simulink model "array_and_Darray_doubleRx"  (R2019b)
settings: Solver=VariableStepAuto  StartTime=0.0  StopTime=0.0005  RelTol=1e-3
libraries: fl_lib x54, nesl_utility x34, ee_lib x17, powerlib_meascontrol x5
settings Model: Creator=LRF  LastModifiedBy=LRF

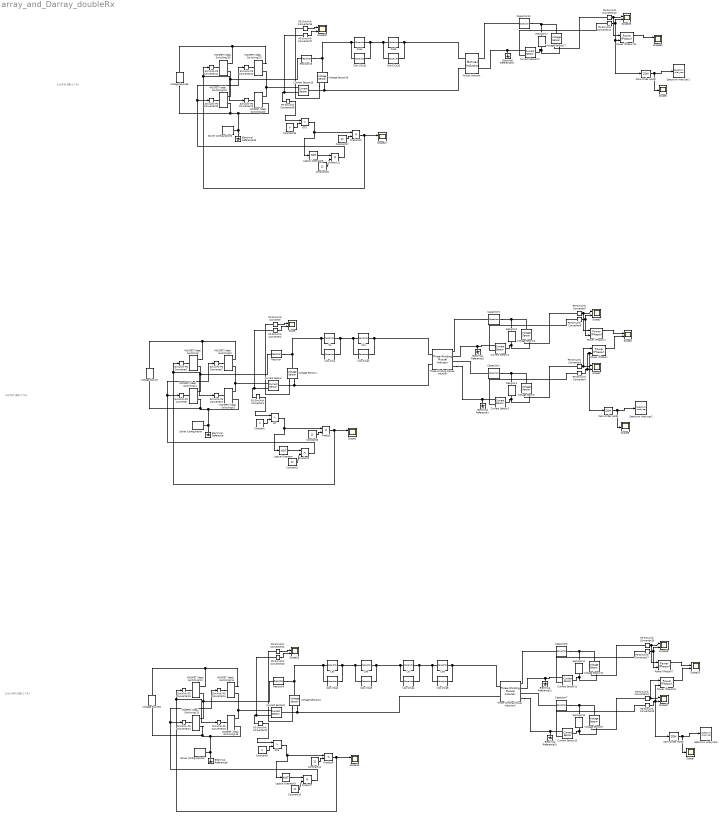
== system array_and_Darray_doubleRx ==
  note: 2x1阵列 搭配 2个Rx
  note: 2x1阵列 搭配 1个Rx
  note: 2x2x1阵列 搭配 2个Rx
  (2/a-1)Ca{,1..5,11..12} (8 alike) : fl_lib/Electrical/Electrical Elements/Capacitor  c=379 pF  r=1e-6 Ohm  g=0 1/Ohm  i_specify=off  i_priority=None  i=0 A  i_nominal_specify=off  i_nominal_unit=A  i_nominal_value=1  v_specify=off  v_priority=None  v=0 V  v_nominal_specify=off  v_nominal_unit=V  v_nominal_value=1  vc_specify=off  vc_priority=High  vc=0 V  vc_nominal_specify=off  vc_nominal_unit=V  vc_nominal_value=1
  Ca{,1,5..8,14..15} (8 alike) : fl_lib/Electrical/Electrical Elements/Capacitor  c=1517 pF  r=1e-6 Ohm  g=0 1/Ohm  i_specify=off  i_priority=None  i=0 A  i_nominal_specify=off  i_nominal_unit=A  i_nominal_value=1  v_specify=off  v_priority=None  v=0 V  v_nominal_specify=off  v_nominal_unit=V  v_nominal_value=1  vc_specify=off  vc_priority=High  vc=0 V  vc_nominal_specify=off  vc_nominal_unit=V  vc_nominal_value=1
  Capacitor{1,3,7..8,12} (5 alike) : fl_lib/Electrical/Electrical Elements/Capacitor  c=1013 pF  r=1e-6 Ohm  g=0 1/Ohm  i_specify=off  i_priority=None  i=0 A  i_nominal_specify=off  i_nominal_unit=A  i_nominal_value=1  v_specify=off  v_priority=None  v=0 V  v_nominal_specify=off  v_nominal_unit=V  v_nominal_value=1  vc_specify=off  vc_priority=High  vc=0 V  vc_nominal_specify=off  vc_nominal_unit=V  vc_nominal_value=1
  Constant : Constant  Value=0
  Constant{1,3,10..11,16..17} (6 alike) : Constant  Value=12
  Constant15 : Constant  Value=0
  Constant9 : Constant  Value=0
  Current Sensor{,1..2,9..11,15,17} (8 alike) : fl_lib/Electrical/Electrical Sensors/Current Sensor
  Electrical Reference{,1..2,9..11,15,17} (8 alike) : fl_lib/Electrical/Electrical Elements/Electrical Reference
  GT : RelationalOperator  Operator=>  OutDataTypeStr=boolean  RndMeth=Simplest
  GT3 : RelationalOperator  Operator=>  OutDataTypeStr=boolean  RndMeth=Simplest
  GT5 : RelationalOperator  Operator=>  OutDataTypeStr=boolean  RndMeth=Simplest
  Logical Operator : Logic  Operator=NOT  AllPortsSameDT=off  OutDataTypeStr=boolean
  Logical Operator3 : Logic  Operator=NOT  AllPortsSameDT=off  OutDataTypeStr=boolean
  Logical Operator5 : Logic  Operator=NOT  AllPortsSameDT=off  OutDataTypeStr=boolean
  MOSFET (Ideal, Switching){,1..3,12..15,20..23} (12 alike) : ee_lib/Semiconductors & Converters/MOSFET (Ideal, Switching)  Rds=0.01 Ohm  Goff=1e-6 1/Ohm  Vth=2 V  diode_param=1  diode_Vf=0.8 V  diode_Ron=0.001 Ohm  diode_Goff=1e-5 1/Ohm  diode_C=50e-9 F  diode_iRM=-235 A  diode_iF=300 A  diode_idot=-50 A/us  diode_trr_param=1  diode_trr_factor=3  diode_trr=15 us  diode_Qrr=1500 s*uA  thermal_loss_option=2  Voff=300 V  Tau=1e-4 s  Tj=[298.15, 398.15] K  Iout_scalar=600 A  Eon_scalar=22.86e-3 J  Eoff_scalar=17.14e-3 J  Von_scalar=2.7 V  Iout_data=[0, 10, 50, 100, 200, 400, 600] A  Eon_data=[0, .29, 1.43, 2.86, 5.71, 13.14, 22.86; 0, .57, 2.63, 5.14, 10.29, 20.57, 30.29] * 1e-3 J  Eoff_data=[0, .21, 1.07, 2.14, 4.29, 9.86, 17.14; 0, .43, 1.97, 3.86, 7.71, 15.43, 22.71] * 1e-3 J  Von_data=[0, 1.1, 1.3, 1.45, 1.75, 2.25, 2.7; 0, 1, 1.15, 1.35, 1.7, 2.35, 3] V
      settings: SourceProductName=Simscape Electrical
  Mutual Inductor : fl_lib/Electrical/Electrical Elements/Mutual Inductor  L1=106.94 uH  L2=100 uH  k=0.1  i1_specify=off  i1_priority=High  i1=0 A  i1_nominal_specify=off  i1_nominal_unit=A  i1_nominal_value=1  i2_specify=off  i2_priority=High  i2=0 A  i2_nominal_specify=off  i2_nominal_unit=A  i2_nominal_value=1  v1_specify=off  v1_priority=None  v1=0 V  v1_nominal_specify=off  v1_nominal_unit=V  v1_nominal_value=1  v2_specify=off  v2_priority=None  v2=0 V  v2_nominal_specify=off  v2_nominal_unit=V  v2_nominal_value=1
      settings: SourceProductName=Simscape  SourceProductBaseCode=SS  InternalSimscapePortConfiguration="{\"Bottom\":[],\"Left\":[{\"id\":\"p1\",\"label\":\"1+\",\"type\":\"foundation.electrical.electrical\"},{\"id\":\"n1\",\"label\":\"1-\",\"type\":\"foundation.electrical.electrical\"}],\"Right\":[{\"id\":\"p2\",\"label\":\"2+\",\"type\":\"foundation.electrical.electrical\"},{\"id\":\"n2\",\"label\":\"2-\",\"type\":\"foundation.electrical.electrical\"}],\"Top\":[]}"
  PS-Simulink Converter{,1..6,21..27,35..37,40..41} (19 alike) : nesl_utility/PS-Simulink Converter  PhysicalDomain=network_engine_domain  SubClassName=ps_output  LeftPortType=input  RightPortType=output  PseudoPeriodic=off  Frequencies=[]  Unit=inherit  AffineConversion=off
  Power (Phasor){,1,6..7,11} (5 alike) : powerlib_meascontrol/Measurements/Power (Phasor)
      settings: SourceProductName=Simscape Electrical  SourceProductBaseCode=PS
  Product{,1,6..7,10..11} (6 alike) : Product
  Resistor : fl_lib/Electrical/Electrical Elements/Resistor  R=0 Ohm  i_specify=off  i_priority=None  i=0 A  i_nominal_specify=off  i_nominal_unit=A  i_nominal_value=1  v_specify=off  v_priority=None  v=0 V  v_nominal_specify=off  v_nominal_unit=V  v_nominal_value=1
  Resistor{1..2,10..11,17} (5 alike) : fl_lib/Electrical/Electrical Elements/Resistor  R=15 Ohm  i_specify=off  i_priority=None  i=0 A  i_nominal_specify=off  i_nominal_unit=A  i_nominal_value=1  v_specify=off  v_priority=None  v=0 V  v_nominal_specify=off  v_nominal_unit=V  v_nominal_value=1
  Resistor15 : fl_lib/Electrical/Electrical Elements/Resistor  R=0 Ohm  i_specify=off  i_priority=None  i=0 A  i_nominal_specify=off  i_nominal_unit=A  i_nominal_value=1  v_specify=off  v_priority=None  v=0 V  v_nominal_specify=off  v_nominal_unit=V  v_nominal_value=1
  Resistor9 : fl_lib/Electrical/Electrical Elements/Resistor  R=0 Ohm  i_specify=off  i_priority=None  i=0 A  i_nominal_specify=off  i_nominal_unit=A  i_nominal_value=1  v_specify=off  v_priority=None  v=0 V  v_nominal_specify=off  v_nominal_unit=V  v_nominal_value=1
  Scope{,1..4,15..19,26..27,29..30} (14 alike) : Scope  NumInputPorts=2
  Scope5 : Scope
  Scope6 : Scope
  Scope7 : Scope
  Simulink-PS Converter{,1..3,12..15,20..23} (12 alike) : nesl_utility/Simulink-PS Converter  PhysicalDomain=network_engine_domain  SubClassName=ps_input  LeftPortType=input  RightPortType=output  PseudoPeriodic=off  Frequencies=[]  NoiseDistribution=none  NoiseParameters=[]  Unit=1  AffineConversion=off  FilteringAndDerivatives=provide  SimscapeFilterOrder=1  InputFilterTimeConstant=0.001  UdotUserProvided=0
  Solver Configuration : nesl_utility/Solver Configuration  PhysicalDomain=network_engine_domain  SubClassName=solver  LeftPortType=input  RightPortType=generic  Tones=[]  Harmonics=[]  SimulateNoise=off  Profile=off  UseLocalSampling=off  EnableSwitchedLinearOptims=on  FrequencyDomain=off  UseCCode=off  RelTol=0.001  AbsTol=1e-06  MinStep=1e-09  ToWorkspace=off  RevertToSquareIcSolve=off  NumHomotopyIterations=100  PhasorMode=off  PhasorModeNumHarmonics=1  DoDC=off  ResidualTolerance=1e-09  UseLocalSolver=off  LocalSolverChoice=NE_BACKWARD_EULER_ADVANCER  LocalSolverSampleTime=0.001  DoFixedCost=off  MaxNonlinIter=3  MaxModeIter=2  LinearAlgebra=auto  EquationFormulation=NE_TIME_EF  DelaysMemoryBudget=1024  AutomaticFiltering=on  FilteringTimeConstant=0.001  PartitionStorageMethod=AS_NEEDED  PartitionMemoryBudget=1024  PartitionMethod=ROBUST
  Solver Configuration3 : nesl_utility/Solver Configuration  PhysicalDomain=network_engine_domain  SubClassName=solver  LeftPortType=input  RightPortType=generic  Tones=[]  Harmonics=[]  SimulateNoise=off  Profile=off  UseLocalSampling=off  EnableSwitchedLinearOptims=on  FrequencyDomain=off  UseCCode=off  RelTol=0.001  AbsTol=1e-06  MinStep=1e-09  ToWorkspace=off  RevertToSquareIcSolve=off  NumHomotopyIterations=100  PhasorMode=off  PhasorModeNumHarmonics=1  DoDC=off  ResidualTolerance=1e-09  UseLocalSolver=off  LocalSolverChoice=NE_BACKWARD_EULER_ADVANCER  LocalSolverSampleTime=0.001  DoFixedCost=off  MaxNonlinIter=3  MaxModeIter=2  LinearAlgebra=auto  EquationFormulation=NE_TIME_EF  DelaysMemoryBudget=1024  AutomaticFiltering=on  FilteringTimeConstant=0.001  PartitionStorageMethod=AS_NEEDED  PartitionMemoryBudget=1024  PartitionMethod=ROBUST
  Solver Configuration5 : nesl_utility/Solver Configuration  PhysicalDomain=network_engine_domain  SubClassName=solver  LeftPortType=input  RightPortType=generic  Tones=[]  Harmonics=[]  SimulateNoise=off  Profile=off  UseLocalSampling=off  EnableSwitchedLinearOptims=on  FrequencyDomain=off  UseCCode=off  RelTol=0.001  AbsTol=1e-06  MinStep=1e-09  ToWorkspace=off  RevertToSquareIcSolve=off  NumHomotopyIterations=100  PhasorMode=off  PhasorModeNumHarmonics=1  DoDC=off  ResidualTolerance=1e-09  UseLocalSolver=off  LocalSolverChoice=NE_BACKWARD_EULER_ADVANCER  LocalSolverSampleTime=0.001  DoFixedCost=off  MaxNonlinIter=3  MaxModeIter=2  LinearAlgebra=auto  EquationFormulation=NE_TIME_EF  DelaysMemoryBudget=1024  AutomaticFiltering=on  FilteringTimeConstant=0.001  PartitionStorageMethod=AS_NEEDED  PartitionMemoryBudget=1024  PartitionMethod=ROBUST
  Spectrum Analyzer1 : SpectrumAnalyzer
  Spectrum Analyzer2 : SpectrumAnalyzer
  Spectrum Analyzer3 : SpectrumAnalyzer
  Three-Winding Mutual Inductor : ee_lib/Passive/Transformers/Three-Winding Mutual Inductor  L1=106.94 uH  L2=100 uH  L3=100 uH  K12=0.1  K13=0.1  K23=0  IC_given=1  IC1=0 A  IC2=0 A  IC3=0 A
      settings: SourceProductName=Simscape Electrical  SourceProductBaseCode=PS  InternalSimscapePortConfiguration="{\"Bottom\":[],\"Left\":[{\"id\":\"p1\",\"label\":\"1+\",\"type\":\"foundation.electrical.electrical\"},{\"id\":\"n1\",\"label\":\"1-\",\"type\":\"foundation.electrical.electrical\"}],\"Right\":[{\"id\":\"p2\",\"label\":\"2+\",\"type\":\"foundation.electrical.electrical\"},{\"id\":\"n2\",\"label\":\"2-\",\"type\":\"foundation.electrical.electrical\"},{\"id\":\"p3\",\"label\":\"3+\",\"type\":\"foundation.electrical.electrical\"},{\"id\":\"n3\",\"label\":\"3-\",\"type\":\"foundation.electrical.electrical\"}],\"Top\":[]}"
  Three-Winding Mutual Inductor3 : ee_lib/Passive/Transformers/Three-Winding Mutual Inductor  L1=213.88 uH  L2=100 uH  L3=100 uH  K12=0.1  K13=0.1  K23=0  IC_given=1  IC1=0 A  IC2=0 A  IC3=0 A
      settings: SourceProductName=Simscape Electrical  SourceProductBaseCode=PS  InternalSimscapePortConfiguration="{\"Bottom\":[],\"Left\":[{\"id\":\"p1\",\"label\":\"1+\",\"type\":\"foundation.electrical.electrical\"},{\"id\":\"n1\",\"label\":\"1-\",\"type\":\"foundation.electrical.electrical\"}],\"Right\":[{\"id\":\"p2\",\"label\":\"2+\",\"type\":\"foundation.electrical.electrical\"},{\"id\":\"n2\",\"label\":\"2-\",\"type\":\"foundation.electrical.electrical\"},{\"id\":\"p3\",\"label\":\"3+\",\"type\":\"foundation.electrical.electrical\"},{\"id\":\"n3\",\"label\":\"3-\",\"type\":\"foundation.electrical.electrical\"}],\"Top\":[]}"
  Voltage Sensor{,1..2,9..11,16..17} (8 alike) : fl_lib/Electrical/Electrical Sensors/Voltage Sensor
  Voltage Source : ee_lib/Sources/Voltage Source  dc_voltage=15 V  ac_voltage=0 V  ac_shift=0 rad  ac_frequency=60 Hz  noise_mode=0  PSD=0 V^2/Hz  repeatability=1  auto_seed=3646982598  user_seed=0  sample_time=1e-3 s  i_specify=off  i_priority=None  i=0 A  i_nominal_specify=off  i_nominal_unit=A  i_nominal_value=1  v_specify=off  v_priority=None  v=0 V  v_nominal_specify=off  v_nominal_unit=V  v_nominal_value=1
      settings: SourceProductName=Simscape Electrical
  Voltage Source3 : ee_lib/Sources/Voltage Source  dc_voltage=15 V  ac_voltage=0 V  ac_shift=0 rad  ac_frequency=60 Hz  noise_mode=0  PSD=0 V^2/Hz  repeatability=1  auto_seed=3181899151  user_seed=0  sample_time=1e-3 s  i_specify=off  i_priority=None  i=0 A  i_nominal_specify=off  i_nominal_unit=A  i_nominal_value=1  v_specify=off  v_priority=None  v=0 V  v_nominal_specify=off  v_nominal_unit=V  v_nominal_value=1
      settings: SourceProductName=Simscape Electrical
  Voltage Source5 : ee_lib/Sources/Voltage Source  dc_voltage=15 V  ac_voltage=0 V  ac_shift=0 rad  ac_frequency=60 Hz  noise_mode=0  PSD=0 V^2/Hz  repeatability=1  auto_seed=2586388248  user_seed=0  sample_time=1e-3 s  i_specify=off  i_priority=None  i=0 A  i_nominal_specify=off  i_nominal_unit=A  i_nominal_value=1  v_specify=off  v_priority=None  v=0 V  v_nominal_specify=off  v_nominal_unit=V  v_nominal_value=1
      settings: SourceProductName=Simscape Electrical
  Zero-Order Hold1 : ZeroOrderHold  SampleTime=1e-7
  Zero-Order Hold2 : ZeroOrderHold  SampleTime=1e-7
  Zero-Order Hold3 : ZeroOrderHold  SampleTime=1e-7
  wires:
  PS-Simulink Converter/1 -> Scope/1
  PS-Simulink Converter2/1 -> Scope/2
  PS-Simulink Converter1/1 -> GT/1
  Constant/1 -> GT/2
  GT/1 -> Logical Operator/1, Product/1
  Product/1 -> Simulink-PS Converter3/1, Simulink-PS Converter1/1, Scope1/1
  Constant3/1 -> Product/2
  Logical Operator/1 -> Product1/1
  Constant1/1 -> Product1/2
  Product1/1 -> Simulink-PS Converter2/1, Simulink-PS Converter/1
  PS-Simulink Converter3/1 -> Power (Phasor)/1, Scope2/1
  PS-Simulink Converter6/1 -> Power (Phasor)1/2, Scope3/2
  PS-Simulink Converter5/1 -> Power (Phasor)1/1, Scope3/1
  Power (Phasor)/1 -> Scope4/2
  Power (Phasor)1/1 -> Scope4/1
  PS-Simulink Converter21/1 -> Scope15/1
  PS-Simulink Converter23/1 -> Scope15/2
  PS-Simulink Converter22/1 -> GT3/1
  PS-Simulink Converter27/1 -> Power (Phasor)7/2, Scope18/2
  Power (Phasor)6/1 -> Scope19/2
  GT3/1 -> Logical Operator3/1, Product6/1
  PS-Simulink Converter24/1 -> Power (Phasor)6/1, Scope17/1
  Product6/1 -> Simulink-PS Converter15/1, Simulink-PS Converter13/1, Scope16/1
  Logical Operator3/1 -> Product7/1
  Product7/1 -> Simulink-PS Converter14/1, Simulink-PS Converter12/1
  Constant9/1 -> GT3/2
  Power (Phasor)7/1 -> Scope19/1
  Constant11/1 -> Product6/2
  Constant10/1 -> Product7/2
  PS-Simulink Converter26/1 -> Power (Phasor)7/1, Scope18/1
  PS-Simulink Converter35/1 -> Scope26/1
  PS-Simulink Converter37/1 -> Scope26/2
  PS-Simulink Converter36/1 -> GT5/1
  GT5/1 -> Logical Operator5/1, Product10/1
  Product10/1 -> Simulink-PS Converter23/1, Simulink-PS Converter21/1, Scope27/1
  Logical Operator5/1 -> Product11/1
  Product11/1 -> Simulink-PS Converter22/1, Simulink-PS Converter20/1
  Constant15/1 -> GT5/2
  Power (Phasor)11/1 -> Scope30/1
  Constant17/1 -> Product10/2
  Constant16/1 -> Product11/2
  PS-Simulink Converter40/1 -> Power (Phasor)11/1, Scope29/1
  PS-Simulink Converter41/1 -> Zero-Order Hold2/1, Power (Phasor)11/2, Scope29/2
  Zero-Order Hold2/1 -> Scope5/1, Spectrum Analyzer1/1
  Zero-Order Hold1/1 -> Scope6/1, Spectrum Analyzer2/1
  PS-Simulink Converter4/1 -> Zero-Order Hold1/1, Power (Phasor)/2, Scope2/2
  PS-Simulink Converter25/1 -> Zero-Order Hold3/1, Power (Phasor)6/2, Scope17/2
  Zero-Order Hold3/1 -> Scope7/1, Spectrum Analyzer3/1
  connections:
  Electrical Reference1/LConn1 -- Three-Winding Mutual Inductor/RConn4 -- Current Sensor1/RConn2
  Capacitor1/RConn1 -- Voltage Sensor/LConn1 -- Resistor1/LConn1
  Capacitor1/LConn1 -- Three-Winding Mutual Inductor/RConn3
  Resistor/RConn1 -- (2/a-1)Ca/LConn1 -- Ca/LConn1 -- Voltage Sensor1/LConn1
  "MOSFET (Ideal, Switching)"/RConn1 -- Voltage Source/LConn1 -- "MOSFET (Ideal, Switching)2"/RConn1
  "MOSFET (Ideal, Switching)1"/RConn1 -- "MOSFET (Ideal, Switching)"/RConn2 -- Resistor/LConn1
  "MOSFET (Ideal, Switching)3"/RConn1 -- Current Sensor/RConn2 -- "MOSFET (Ideal, Switching)2"/RConn2
  "MOSFET (Ideal, Switching)1"/RConn2 -- Voltage Source/RConn1 -- Solver Configuration/RConn1 -- Electrical Reference/LConn1 -- "MOSFET (Ideal, Switching)3"/RConn2
  Simulink-PS Converter/RConn1 -- "MOSFET (Ideal, Switching)1"/LConn1
  Simulink-PS Converter1/RConn1 -- "MOSFET (Ideal, Switching)"/LConn1
  Simulink-PS Converter2/RConn1 -- "MOSFET (Ideal, Switching)2"/LConn1
  Simulink-PS Converter3/RConn1 -- "MOSFET (Ideal, Switching)3"/LConn1
  Voltage Sensor1/RConn2 -- Three-Winding Mutual Inductor/LConn2 -- Current Sensor/LConn1
  Current Sensor/RConn1 -- PS-Simulink Converter2/LConn1 -- PS-Simulink Converter1/LConn1
  Voltage Sensor/RConn2 -- Current Sensor1/LConn1 -- Resistor1/RConn1
  Voltage Sensor1/RConn1 -- PS-Simulink Converter/LConn1
  PS-Simulink Converter3/LConn1 -- Voltage Sensor/RConn1
  Current Sensor1/RConn1 -- PS-Simulink Converter4/LConn1
  Resistor2/RConn1 -- Voltage Sensor2/RConn2 -- Current Sensor2/LConn1
  Current Sensor2/RConn2 -- Electrical Reference2/LConn1 -- Three-Winding Mutual Inductor/RConn2
  Resistor2/LConn1 -- Capacitor3/RConn1 -- Voltage Sensor2/LConn1
  Capacitor3/LConn1 -- Three-Winding Mutual Inductor/RConn1
  PS-Simulink Converter5/LConn1 -- Voltage Sensor2/RConn1
  Current Sensor2/RConn1 -- PS-Simulink Converter6/LConn1
  (2/a-1)Ca/RConn1 -- (2/a-1)Ca1/LConn1 -- Ca1/LConn1 -- Ca/RConn1
  (2/a-1)Ca1/RConn1 -- Three-Winding Mutual Inductor/LConn1 -- Ca1/RConn1
  (2/a-1)Ca4/LConn1 -- Ca7/LConn1 -- Ca6/RConn1 -- (2/a-1)Ca3/RConn1
  Current Sensor10/RConn2 -- Electrical Reference10/LConn1 -- Three-Winding Mutual Inductor3/RConn4
  Three-Winding Mutual Inductor3/RConn2 -- Current Sensor11/RConn2 -- Electrical Reference11/LConn1
  Resistor10/LConn1 -- Capacitor7/RConn1 -- Voltage Sensor9/LConn1
  Voltage Sensor10/LConn1 -- Resistor9/RConn1 -- (2/a-1)Ca2/LConn1 -- Ca5/LConn1
  Current Sensor11/LConn1 -- Resistor11/RConn1 -- Voltage Sensor11/RConn2
  "MOSFET (Ideal, Switching)14"/RConn1 -- "MOSFET (Ideal, Switching)12"/RConn1 -- Voltage Source3/LConn1
  "MOSFET (Ideal, Switching)14"/RConn2 -- "MOSFET (Ideal, Switching)15"/RConn1 -- Current Sensor9/RConn2
  Ca5/RConn1 -- (2/a-1)Ca2/RConn1 -- (2/a-1)Ca3/LConn1 -- Ca6/LConn1
  Resistor9/LConn1 -- "MOSFET (Ideal, Switching)13"/RConn1 -- "MOSFET (Ideal, Switching)12"/RConn2
  PS-Simulink Converter22/LConn1 -- Current Sensor9/RConn1 -- PS-Simulink Converter23/LConn1
  Voltage Sensor11/LConn1 -- Resistor11/LConn1 -- Capacitor8/RConn1
  Current Sensor9/LConn1 -- Voltage Sensor10/RConn2 -- Three-Winding Mutual Inductor3/LConn2
  "MOSFET (Ideal, Switching)15"/RConn2 -- Solver Configuration3/RConn1 -- Electrical Reference9/LConn1 -- "MOSFET (Ideal, Switching)13"/RConn2 -- Voltage Source3/RConn1
  Resistor10/RConn1 -- Voltage Sensor9/RConn2 -- Current Sensor10/LConn1
  Capacitor8/LConn1 -- Three-Winding Mutual Inductor3/RConn1
  PS-Simulink Converter26/LConn1 -- Voltage Sensor11/RConn1
  Simulink-PS Converter13/RConn1 -- "MOSFET (Ideal, Switching)12"/LConn1
  Capacitor7/LConn1 -- Three-Winding Mutual Inductor3/RConn3
  Current Sensor10/RConn1 -- PS-Simulink Converter25/LConn1
  Simulink-PS Converter15/RConn1 -- "MOSFET (Ideal, Switching)15"/LConn1
  Simulink-PS Converter14/RConn1 -- "MOSFET (Ideal, Switching)14"/LConn1
  Current Sensor11/RConn1 -- PS-Simulink Converter27/LConn1
  PS-Simulink Converter24/LConn1 -- Voltage Sensor9/RConn1
  Voltage Sensor10/RConn1 -- PS-Simulink Converter21/LConn1
  Simulink-PS Converter12/RConn1 -- "MOSFET (Ideal, Switching)13"/LConn1
  Ca8/LConn1 -- (2/a-1)Ca5/LConn1 -- (2/a-1)Ca4/RConn1 -- Ca7/RConn1
  (2/a-1)Ca5/RConn1 -- Three-Winding Mutual Inductor3/LConn1 -- Ca8/RConn1
  Ca15/RConn1 -- Mutual Inductor/LConn1 -- (2/a-1)Ca12/RConn1
  Electrical Reference17/LConn1 -- Mutual Inductor/RConn2 -- Current Sensor17/RConn2
  Voltage Sensor16/LConn1 -- Resistor15/RConn1 -- (2/a-1)Ca11/LConn1 -- Ca14/LConn1
  Current Sensor17/LConn1 -- Resistor17/RConn1 -- Voltage Sensor17/RConn2
  "MOSFET (Ideal, Switching)22"/RConn1 -- "MOSFET (Ideal, Switching)20"/RConn1 -- Voltage Source5/LConn1
  "MOSFET (Ideal, Switching)22"/RConn2 -- "MOSFET (Ideal, Switching)23"/RConn1 -- Current Sensor15/RConn2
  Ca14/RConn1 -- (2/a-1)Ca11/RConn1 -- (2/a-1)Ca12/LConn1 -- Ca15/LConn1
  Resistor15/LConn1 -- "MOSFET (Ideal, Switching)21"/RConn1 -- "MOSFET (Ideal, Switching)20"/RConn2
  PS-Simulink Converter36/LConn1 -- Current Sensor15/RConn1 -- PS-Simulink Converter37/LConn1
  Voltage Sensor17/LConn1 -- Resistor17/LConn1 -- Capacitor12/RConn1
  Current Sensor15/LConn1 -- Mutual Inductor/LConn2 -- Voltage Sensor16/RConn2
  "MOSFET (Ideal, Switching)23"/RConn2 -- Solver Configuration5/RConn1 -- Electrical Reference15/LConn1 -- "MOSFET (Ideal, Switching)21"/RConn2 -- Voltage Source5/RConn1
  Capacitor12/LConn1 -- Mutual Inductor/RConn1
  PS-Simulink Converter40/LConn1 -- Voltage Sensor17/RConn1
  Simulink-PS Converter21/RConn1 -- "MOSFET (Ideal, Switching)20"/LConn1
  Simulink-PS Converter20/RConn1 -- "MOSFET (Ideal, Switching)21"/LConn1
  Simulink-PS Converter23/RConn1 -- "MOSFET (Ideal, Switching)23"/LConn1
  Simulink-PS Converter22/RConn1 -- "MOSFET (Ideal, Switching)22"/LConn1
  Voltage Sensor16/RConn1 -- PS-Simulink Converter35/LConn1
  Current Sensor17/RConn1 -- PS-Simulink Converter41/LConn1
